simulink model "battery_cell_balancing_comparison"  (R2024b)
settings: Solver=FixedStepAuto  StartTime=0.0  StopTime=18000  FixedStep=0.05  RelTol=1e-4
PostLoadFcn:
  | open('C:\GitHub\module_ecm_analysis\battery_cell_balancing_initialisation.m');
  | run('C:\GitHub\module_ecm_analysis\battery_cell_balancing_initialisation.m');
values from neighbouring files (symbols this model uses):
  first_pol_res = ((first_pol_res_charge + first_pol_res_discharge)/2)    [battery_block_initialisation.m]    (also in battery_cell_balancing_initialisation.m; battery_module_hppc_initialisation.m)
  ocv_net = (ocv_charge + ocv_discharge)*12/2    [battery_block_initialisation.m]    (also in battery_cell_balancing_initialisation.m; battery_module_hppc_initialisation.m)
  ohmic_res_charge = [6.498281089,5.36625,4.38375,4.21925 ... (first row only)    [battery_block_initialisation.m]    (also in battery_cell_balancing_initialisation.m; battery_module_hppc_initialisation.m)
  ohmic_res_discharge = [6.556865079,5.427333333,4.425111111,4.245777778 ... (first row only)    [battery_block_initialisation.m]    (also in battery_cell_balancing_initialisation.m; battery_module_hppc_initialisation.m)
  second_pol_res = [4.604829812,6.347286942,4.126604008,2.619409304 ... (first row only)    [battery_block_initialisation.m]    (also in battery_cell_balancing_initialisation.m; battery_module_hppc_initialisation.m; empirical_ecm_initialisation.m)
  soc_init = 0.9*ones(1,16)    [battery_block_initialisation.m]    (also in battery_module_hppc_initialisation.m)
  term_volt = [3.52714940619431 ... (first row only)    [battery_cell_balancing_initialisation.m]
libraries: nesl_utility x216, fl_lib x168, ee_lib x60, batteryecm_lib x48, simulink x3
(part 4 of 4)

== matlab function battery_cell_balancing_comparison/balancing1 ==
  data: pack_current input; cell_voltages input; cell_bal_cmd output
  events: trigger input RISING_EDGE_EVENT
function cell_bal_cmd = balancing(pack_current, cell_voltages)
%cell_bal_cmd = Simulink.Bus.createMATLABStruct('cell_bal_bus');

min_cell_volt = min(cell_voltages);
if abs(pack_current) < 20
    cell_bal_cmd = boolean(cell_voltages > (min_cell_volt + 0.02));
else
    cell_bal_cmd = boolean(zeros(length(cell_voltages),1));
end

end

== matlab function battery_cell_balancing_comparison/balancing5 ==
  data: pack_current input; cell_voltages input; cell_bal_cmd output
  events: trigger input RISING_EDGE_EVENT
function cell_bal_cmd = balancing(pack_current, cell_voltages)
%cell_bal_cmd = Simulink.Bus.createMATLABStruct('cell_bal_bus');

min_cell_volt = min(cell_voltages);
if abs(pack_current) < 20
    cell_bal_cmd = boolean(cell_voltages > (min_cell_volt + 0.02));
else
    cell_bal_cmd = boolean(zeros(length(cell_voltages),1));
end

end

== matlab function battery_cell_balancing_comparison/balancing2 ==
  data: pack_current input; cell_voltages input; cell_bal_cmd output
  events: trigger input RISING_EDGE_EVENT
function cell_bal_cmd = balancing(pack_current, cell_voltages)
%cell_bal_cmd = Simulink.Bus.createMATLABStruct('cell_bal_bus');

min_cell_volt = min(cell_voltages);
if abs(pack_current) < 0.01
    cell_bal_cmd = boolean(cell_voltages > (min_cell_volt + 0.01));
else
    cell_bal_cmd = boolean(zeros(length(cell_voltages),1));
end

end

== matlab function battery_cell_balancing_comparison/balancing3 ==
  data: pack_current input; cell_voltages input; cell_bal_cmd output
  events: trigger input RISING_EDGE_EVENT
function cell_bal_cmd = balancing(pack_current, cell_voltages)
%cell_bal_cmd = Simulink.Bus.createMATLABStruct('cell_bal_bus');

min_cell_volt = min(cell_voltages);
if abs(pack_current) < 20
    cell_bal_cmd = boolean(cell_voltages > (min_cell_volt + 0.02));
else
    cell_bal_cmd = boolean(zeros(length(cell_voltages),1));
end

end
